simulink model "a6nl_sw_modelworkspace_lsg"  (R2018b)
settings: Solver=ode45  StartTime=0.0  StopTime=10.0  MaxStep=0.01  RelTol=1e-3  EnableMultiTasking=on
model workspace (MAT data in the model file):
  c = 4
  k = 1
  m = 2
  v0 = 0
  y0 = 3
settings Model: Creator=Reichl  LastModifiedBy=Reichl
settings DataIOCC: LimitDataPoints=on  SaveFormat=Array  SignalLoggingSaveFormat=ModelDataLogs
settings OptimizationCC: ExpressionDepthLimit=2147483647  LifeSpan=inf
settings DebuggingCC: UnderspecifiedInitializationDetection=Classic  MergeDetectMultiDrivingBlocksExec=none  SolverPrmCheckMsg=warning  FcnCallInpInsideContextMsg=warning  StateNameClashWarn=warning  SFUnexpectedBacktrackingDiag=warning  SFNoUnconditionalDefaultTransitionDiag=warning  SFExecutionAtInitializationDiag=none
settings HardwareCC: ProdBitPerPointer=32  ProdBitPerSizeT=32  ProdBitPerPtrDiffT=32  ProdLargestAtomicFloat=None  ProdIntDivRoundTo=Undefined  ProdEndianess=Unspecified  ProdWordSize=32  ProdHWDeviceType=32-bit Generic
settings ModelReferenceCC: PropagateSignalLabelsOutOfModel=off
settings SFSimCC: SimUseLocalCustomCode=off
settings RTWCC: RTWUseLocalCustomCode=off
settings CodeAppCC: StateflowObjectComments=on
settings GRTTargetCC: TargetLangStandard=C89/C90 (ANSI)  GeneratePreprocessorConditionals=Disable all  CombineOutputUpdateFcns=off  GRTInterface=on
settings ConfigComp: CovMetricSettings=dw  CovHtmlReporting=on  CovSaveCumulativeToWorkspaceVar=on  CovSaveSingleToWorkspaceVar=on  CovExternalEMLEnable=off  CovSFcnEnable=off

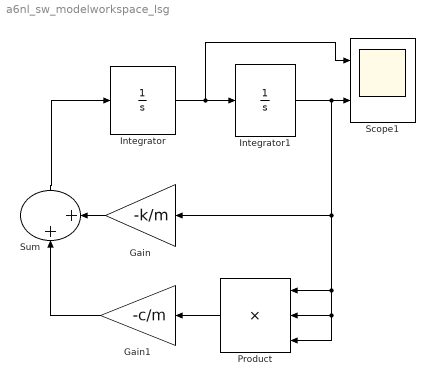
== system a6nl_sw_modelworkspace_lsg ==
  Gain : Gain  Gain=-k/m
  Gain1 : Gain  Gain=-c/m
  Integrator : Integrator  InitialCondition=v0
  Integrator1 : Integrator  InitialCondition=y0
  Product : Product  Inputs=***  RndMeth=Zero
  Scope1 : Scope  NumInputPorts=2
  Sum : Sum  Inputs=|++
  wires:
  Integrator/1 -> Integrator1/1, Scope1/1
  Integrator1/1 -> Scope1/2, Product/3, Product/2, Product/1, Gain/1
  Gain/1 -> Sum/2
  Product/1 -> Gain1/1
  Gain1/1 -> Sum/1
  Sum/1 -> Integrator/1
